simulink library "forceGravBuoy"  (R2018b)
settings: Solver=VariableStepAuto  StartTime=0.0  StopTime=10.0  RelTol=1e-3
values from neighbouring files (symbols this model uses):
  g = 9.81    [Platform.m]    (also in sprungODE.m = system_param.g)
  mass = massplatform.Value    [anchorTetherClass.m]
  rho = 1000    [Platform.m]
undefined symbols (not defined in the file or in its folder): volume
settings Model: Creator=embeato2  LastModifiedBy=embeato2

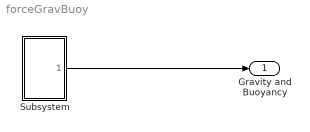
== system forceGravBuoy ==
  Subsystem : Subsystem
  Gravity and Buoyancy : Outport
  wires:
  Subsystem/1(Gravity and Buoyancy) -> Gravity and Buoyancy/1

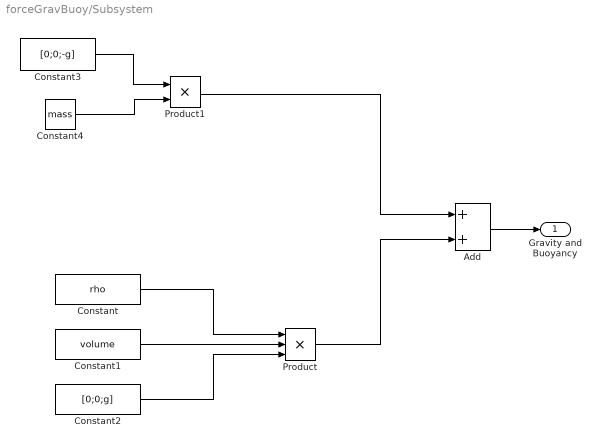
== system forceGravBuoy/Subsystem ==
  Add : Sum
  Constant : Constant  Value=rho
  Constant1 : Constant  Value=volume
  Constant2 : Constant  Value=[0;0;g]
  Constant3 : Constant  Value=[0;0;-g]
  Constant4 : Constant  Value=mass
  Product : Product  Inputs=3
  Product1 : Product
  Gravity and Buoyancy : Outport
  wires:
  Constant4/1 -> Product1/2
  Constant2/1 -> Product/3
  Constant/1 -> Product/1
  Product/1 -> Add/2
  Product1/1 -> Add/1
  Constant1/1 -> Product/2
  Add/1 -> Gravity and Buoyancy/1
  Constant3/1 -> Product1/1
